simulink model "Powersystem_FMU"  (R2022a)
settings: Solver=ode23s  StartTime=0.0  StopTime=10  RelTol=1e-3
settings Model: Creator=au707539  LastModifiedBy=au528638
settings SolverCC: MaxZcPerStep=1

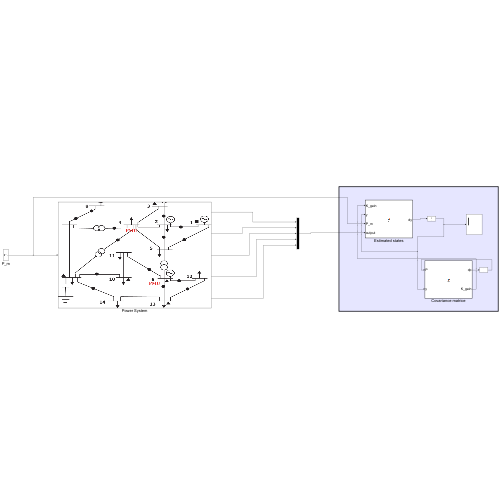
[thumbnail: Simulink's stored preview of the top-level diagram]
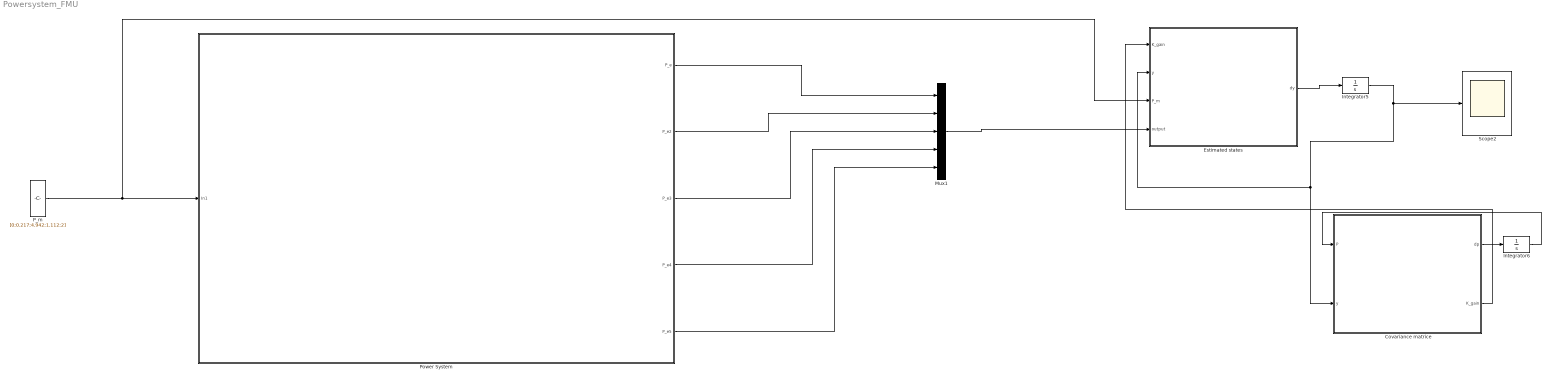
== system Powersystem_FMU ==
  Covariance matrice : MATLAB Function  TreatAsAtomicUnit=on
  Estimated states : MATLAB Function  TreatAsAtomicUnit=on
  Integrator5 : Integrator  InitialCondition=[1.07618884220704,1,0.179610235169918,1,-0.222670000000000,0.951,-0.152730000000000,0.91,-0.230910000000000,1]'
  Integrator6 : Integrator  InitialCondition=1*eye(10)
  Mux1 : Mux  Inputs=5
  P_m : Constant  Value=[0;0.217;4.942;1.112;2]
  Power System : Subsystem
      mask Display: image('IEEE.png'); % Use "Edit Image" on toolstrip to change.
  Scope2 : Scope
  wires:
  P_m/1 -> Estimated states/3(P_m), Power System/1(In1)
  Estimated states/1(dy) -> Integrator5/1
  Integrator5/1 -> Estimated states/2(y), Covariance matrice/2(y), Scope2/1
  Covariance matrice/1(dp) -> Integrator6/1
  Integrator6/1 -> Covariance matrice/1(P)
  Covariance matrice/2(K_gain) -> Estimated states/1(K_gain)
  Mux1/1 -> Estimated states/4(output)
  Power System/1(P_e) -> Mux1/1
  Power System/2(P_e2) -> Mux1/2
  Power System/3(P_e3) -> Mux1/3
  Power System/4(P_e4) -> Mux1/4
  Power System/5(P_e5) -> Mux1/5

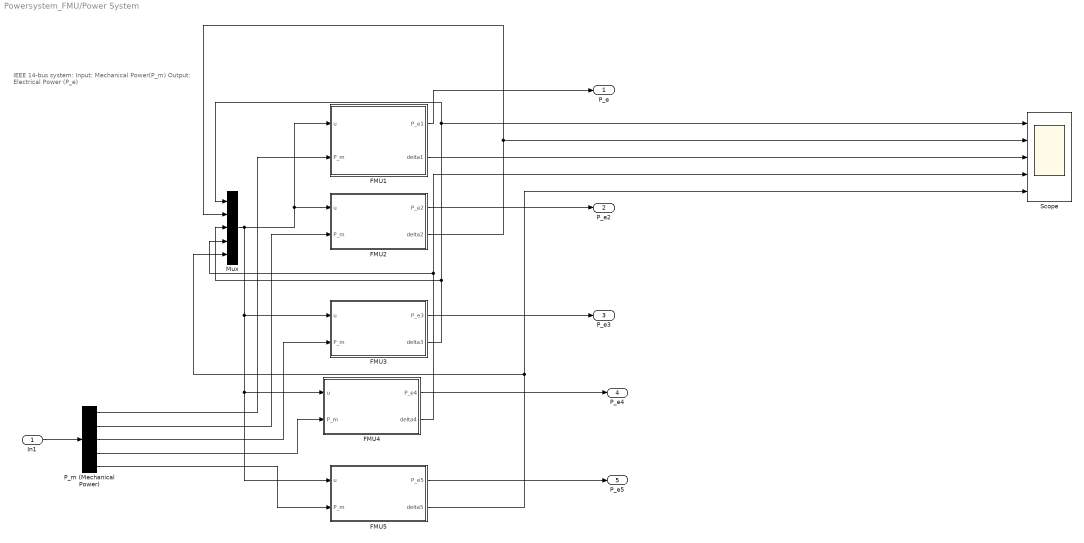
== system Powersystem_FMU/Power System ==
  note: IEEE 14-bus system:
      | Input: Mechanical Power(P_m)
      | Output: Electrical Power (P_e)
  In1 : Inport
  FMU1 : Subsystem
  FMU2 : Subsystem
  FMU3 : Subsystem
  FMU4 : Subsystem
  FMU5 : Subsystem
  Mux : Mux  Inputs=5
  P_m (Mechanical Power) : Demux  Outputs=5
  Scope : Scope  NumInputPorts=5
  P_e : Outport
  P_e2 : Outport  Port=2
  P_e3 : Outport  Port=3
  P_e4 : Outport  Port=4
  P_e5 : Outport  Port=5
  wires:
  FMU1/2(delta1) -> Scope/1, Mux/1
  FMU2/2(delta2) -> Scope/2, Mux/2
  In1/1 -> P_m (Mechanical Power)/1
  P_m (Mechanical Power)/1 -> FMU1/2(P_m)
  FMU1/1(P_e1) -> P_e/1
  P_m (Mechanical Power)/2 -> FMU2/2(P_m)
  FMU2/1(P_e2) -> P_e2/1
  P_m (Mechanical Power)/3 -> FMU3/2(P_m)
  FMU3/2(delta3) -> Scope/3, Mux/3
  FMU3/1(P_e3) -> P_e3/1
  P_m (Mechanical Power)/4 -> FMU4/2(P_m)
  FMU4/2(delta4) -> Scope/4, Mux/4
  FMU4/1(P_e4) -> P_e4/1
  P_m (Mechanical Power)/5 -> FMU5/2(P_m)
  FMU5/1(P_e5) -> P_e5/1
  FMU5/2(delta5) -> Mux/5, Scope/5
  Mux/1 -> FMU5/1(u), FMU4/1(u), FMU3/1(u), FMU2/1(u), FMU1/1(u)

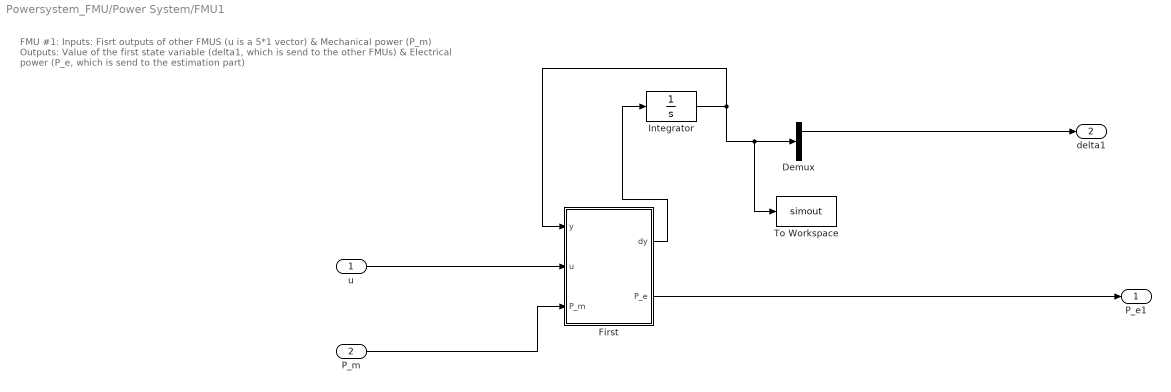
== system Powersystem_FMU/Power System/FMU1 ==
  note: FMU #1:
      | Inputs: Fisrt outputs of other FMUS (u is a 5*1 vector) & Mechanical power (P_m)
      | Outputs: Value of the first state variable (delta1, which is send to the other FMUs) & Electrical power (P_e, which is send to the estimation part)
  u : Inport
  P_m : Inport  Port=2
  Demux : Demux  Outputs=2
  First : MATLAB Function  TreatAsAtomicUnit=on
  Integrator : Integrator  InitialCondition=[1.0762;1]
  To Workspace : ToWorkspace  VariableName=simout  SaveFormat=Timeseries  SampleTime=-1
  P_e1 : Outport
  delta1 : Outport  Port=2
  wires:
  u/1 -> First/2(u)
  Integrator/1 -> First/1(y), To Workspace/1, Demux/1
  First/1(dy) -> Integrator/1
  P_m/1 -> First/3(P_m)
  First/2(P_e) -> P_e1/1
  Demux/1 -> delta1/1

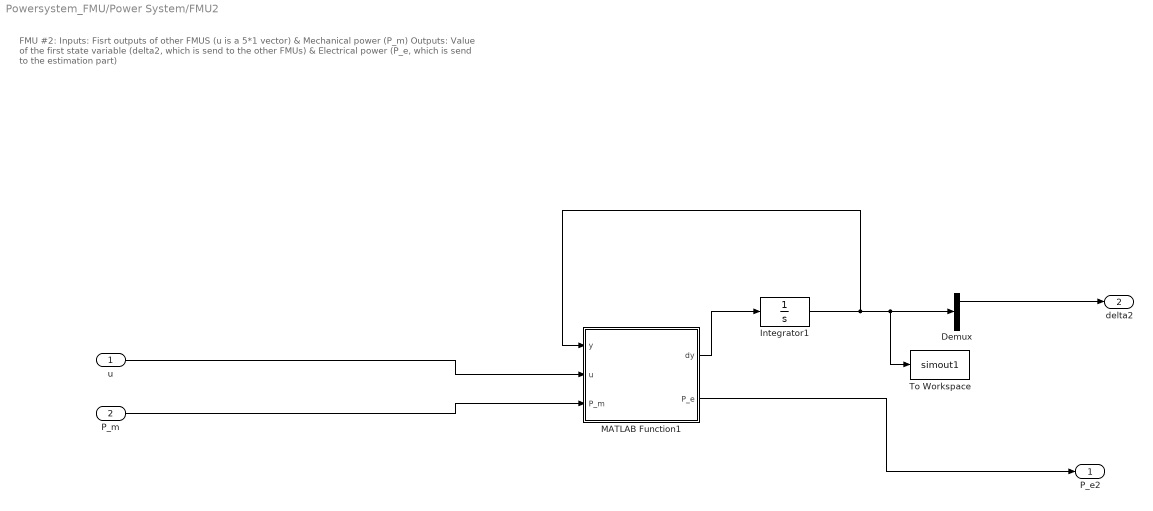
== system Powersystem_FMU/Power System/FMU2 ==
  note: FMU #2:
      | Inputs: Fisrt outputs of other FMUS (u is a 5*1 vector) & Mechanical power (P_m)
      | Outputs: Value of the first state variable (delta2, which is send to the other FMUs) & Electrical power (P_e, which is send to the estimation part)
  u : Inport
  P_m : Inport  Port=2
  Demux : Demux  Outputs=2
  Integrator1 : Integrator  InitialCondition=[0.1796;1]
  MATLAB Function1 : MATLAB Function  TreatAsAtomicUnit=on
  To Workspace : ToWorkspace  VariableName=simout1  SaveFormat=Timeseries  SampleTime=-1
  P_e2 : Outport
  delta2 : Outport  Port=2
  wires:
  P_m/1 -> MATLAB Function1/3(P_m)
  MATLAB Function1/1(dy) -> Integrator1/1
  u/1 -> MATLAB Function1/2(u)
  Integrator1/1 -> To Workspace/1, Demux/1, MATLAB Function1/1(y)
  Demux/1 -> delta2/1
  MATLAB Function1/2(P_e) -> P_e2/1

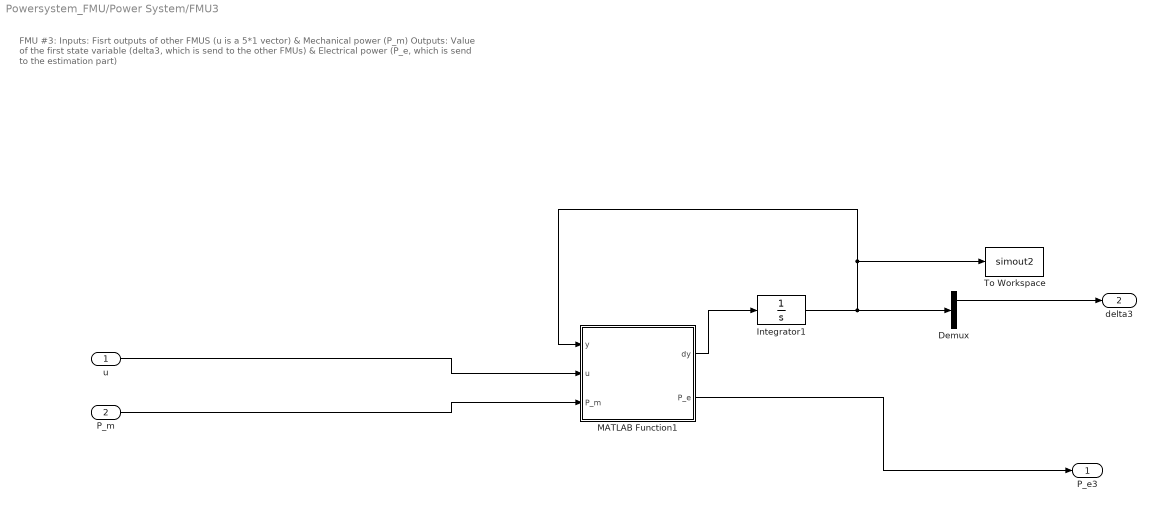
== system Powersystem_FMU/Power System/FMU3 ==
  note: FMU #3:
      | Inputs: Fisrt outputs of other FMUS (u is a 5*1 vector) & Mechanical power (P_m)
      | Outputs: Value of the first state variable (delta3, which is send to the other FMUs) & Electrical power (P_e, which is send to the estimation part)
  u : Inport
  P_m : Inport  Port=2
  Demux : Demux  Outputs=2
  Integrator1 : Integrator  InitialCondition=[0.1796;1]
  MATLAB Function1 : MATLAB Function  TreatAsAtomicUnit=on
  To Workspace : ToWorkspace  VariableName=simout2  SaveFormat=Timeseries  SampleTime=-1
  P_e3 : Outport
  delta3 : Outport  Port=2
  wires:
  P_m/1 -> MATLAB Function1/3(P_m)
  MATLAB Function1/1(dy) -> Integrator1/1
  u/1 -> MATLAB Function1/2(u)
  Integrator1/1 -> Demux/1, To Workspace/1, MATLAB Function1/1(y)
  Demux/1 -> delta3/1
  MATLAB Function1/2(P_e) -> P_e3/1

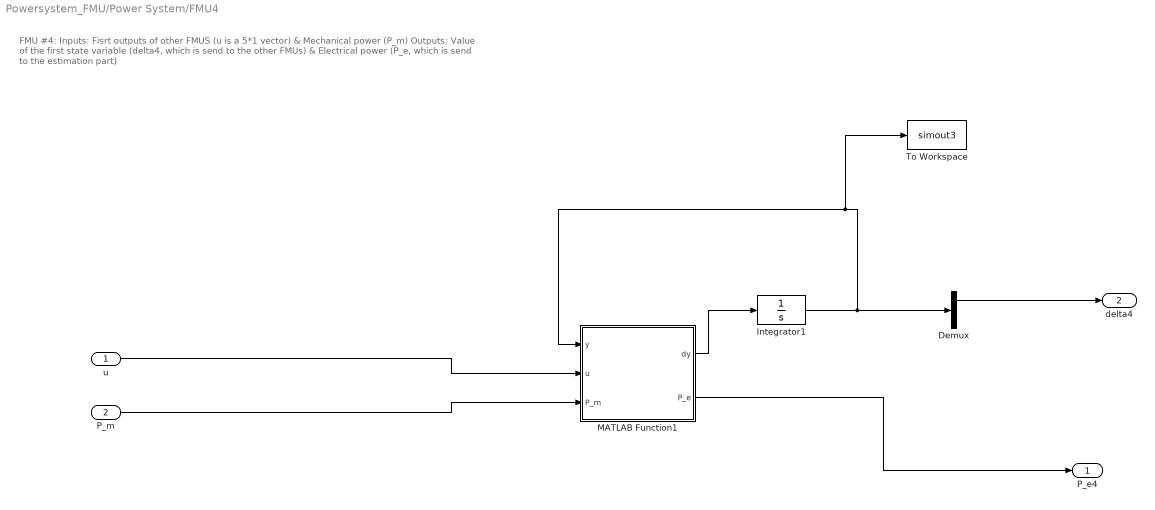
== system Powersystem_FMU/Power System/FMU4 ==
  note: FMU #4:
      | Inputs: Fisrt outputs of other FMUS (u is a 5*1 vector) & Mechanical power (P_m)
      | Outputs: Value of the first state variable (delta4, which is send to the other FMUs) & Electrical power (P_e, which is send to the estimation part)
  u : Inport
  P_m : Inport  Port=2
  Demux : Demux  Outputs=2
  Integrator1 : Integrator  InitialCondition=[0.1796;1]
  MATLAB Function1 : MATLAB Function  TreatAsAtomicUnit=on
  To Workspace : ToWorkspace  VariableName=simout3  SaveFormat=Timeseries  SampleTime=-1
  P_e4 : Outport
  delta4 : Outport  Port=2
  wires:
  P_m/1 -> MATLAB Function1/3(P_m)
  MATLAB Function1/1(dy) -> Integrator1/1
  u/1 -> MATLAB Function1/2(u)
  Demux/1 -> delta4/1
  MATLAB Function1/2(P_e) -> P_e4/1
  Integrator1/1 -> Demux/1, To Workspace/1, MATLAB Function1/1(y)

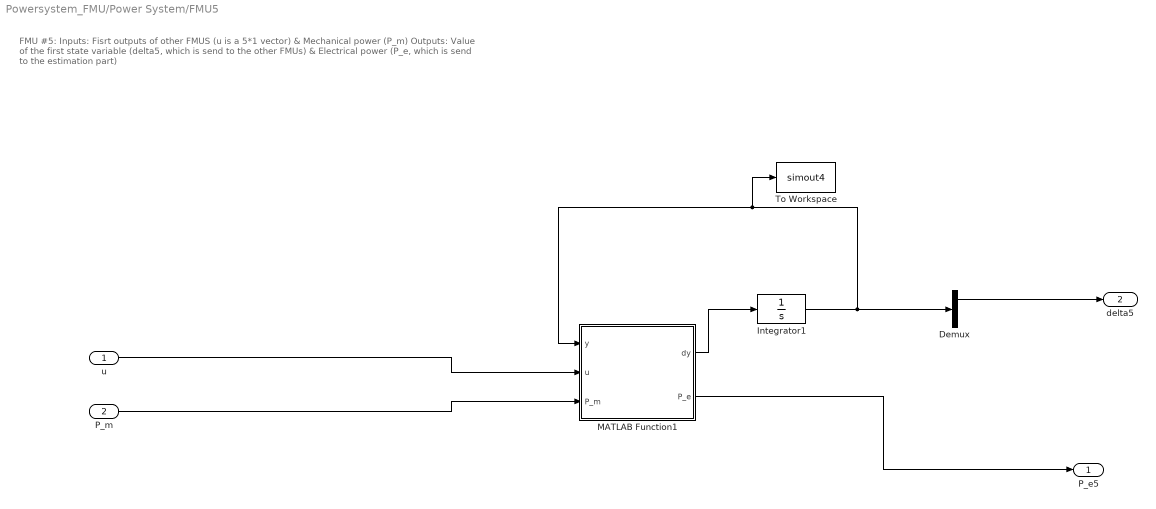
== system Powersystem_FMU/Power System/FMU5 ==
  note: FMU #5:
      | Inputs: Fisrt outputs of other FMUS (u is a 5*1 vector) & Mechanical power (P_m)
      | Outputs: Value of the first state variable (delta5, which is send to the other FMUs) & Electrical power (P_e, which is send to the estimation part)
  u : Inport
  P_m : Inport  Port=2
  Demux : Demux  Outputs=2
  Integrator1 : Integrator  InitialCondition=[0.1796;1]
  MATLAB Function1 : MATLAB Function  TreatAsAtomicUnit=on
  To Workspace : ToWorkspace  VariableName=simout4  SaveFormat=Timeseries  SampleTime=-1
  P_e5 : Outport
  delta5 : Outport  Port=2
  wires:
  P_m/1 -> MATLAB Function1/3(P_m)
  MATLAB Function1/1(dy) -> Integrator1/1
  u/1 -> MATLAB Function1/2(u)
  Integrator1/1 -> Demux/1, To Workspace/1, MATLAB Function1/1(y)
  Demux/1 -> delta5/1
  MATLAB Function1/2(P_e) -> P_e5/1

== matlab function Powersystem_FMU/Power System/FMU2/MATLAB Function1 ==
  data: y input; u input; dy output; P_m input; P_e output
%% This function formulates the dynamic model of the second synchronous machine in IEEE-14 bus test system
%% y is the state vector related to this Genrator, u is vector of all generators angles (delta), and P-m is Mechanical power injected to this machine
%% dy is the derivative of y which is calculated in this function and P-e is the electrical power which is calculated in this function
function [dy,P_e] = fcn(y,u,P_m)
dy=zeros(2,1);
P_e=0;
%%%%%%%Generators and network parameters (they can be defined as global
%%%%%%%parameters because they are fixed for all generators)%%%%%%%%%%%
N_SG=5;
X_d=[0.898 1.05 1.05 1.25 1.25];
Vol_mag=[1.06 1.045 1.01 1.011981 1.049336 1.016012 1.07 1.09 1.032756 1.03177 1.04708 1.053428 1.046967 1.020701];
P_Gen=[2.32 0.4 0 0 0];
Q_Gen=[0 0.424 0 0 0];
VOl_mag_Gen=[Vol_mag(1) Vol_mag(2) Vol_mag(3) Vol_mag(6) Vol_mag(8)];
M=[3.52e-3 0.436e-3 0.436e-3 1.406e-4 1.406e-4];
D=[2 2 2 2 2];
Y=[0.1017-2.4199i, 0.0096+0.9097i, -0.0567+0.5006i, -0.0322+0.4973i, -0.0186+0.5531i; 0.0096+0.9097i, 0.1375-3.5521i, -0.0574+0.9568i, -0.0437+0.8608i, ...
    -0.0395+0.8903i; -0.0567+0.5006i, -0.0574+0.9568i, 0.2630-2.9134i, -0.0640+0.8148i, -0.0791+0.6968i; -0.0322+0.4973i, -0.0437+0.8608i, -0.0640+0.8148i,...
    0.1156-3.0762i, 0.0303+0.9547i; -0.0186+0.5531i, -0.0395+0.8903i, -0.0791+0.6968i, 0.0303+0.9547i, 0.1117-3.0513i];
% [v_r, v_i]=pol2cart(Degrre_Gen,Vol_mag_Gen);

E_abs=zeros(5,1);
for i=1:5
    %     delta0(i)=angle(VOl_mag_Gen(i)+Q_Gen(i).*X_d(i)./VOl_mag_Gen(i) + 1i*P_Gen(i).*X_d(i)./VOl_mag_Gen(i))+Degrre_Gen(i);
    E_abs(i)=abs(VOl_mag_Gen(i)+Q_Gen(i).*X_d(i)./VOl_mag_Gen(i) + 1i*P_Gen(i).*X_d(i)./VOl_mag_Gen(i));
end
%%%%%%%%%%%%%%%%%%%%%%%%%%
delta=u(1:5);
sum1=0; %% local parameter
for j=1:N_SG

    sum1=sum1+E_abs(2)*E_abs(j)*abs(Y(2,j))*cos(delta(2)-delta(j)-angle(Y(2,j))); % All angles in Radian
end
P_e=sum1;

P_e=sum1;  % Second output (which is send to the estimation part)

dy(1)=y(2); %first entry of the function output

dy(2) =(1/M(2))*(P_m-P_e-D(2)*y(2));  %Second entry of the function output

== matlab function Powersystem_FMU/Power System/FMU1/First ==
  data: y input; u input; dy output; P_m input; P_e output
%% This function formulates the dynamic model of the first synchronous machine in IEEE-14 bus test system
%% y is the state vector related to this Genrator, u is vector of all generators angles (delta), and P-m is Mechanical power injected to this machine
%% dy is the derivative of y which is calculated in this function and P-e is the electrical power which is calculated in this function
function [dy,P_e] = fcn(y,u,P_m) 
dy=zeros(2,1);

%%%%%%%Generators and network parameters (they can be defined as global
%%%%%%%parameters because they are fixed for all generators)%%%%%%%%%%%%%
N_SG=5;
X_d=[0.898 1.05 1.05 1.25 1.25];
Vol_mag=[1.06 1.045 1.01 1.011981 1.049336 1.016012 1.07 1.09 1.032756 1.03177 1.04708 1.053428 1.046967 1.020701];
P_Gen=[2.32 0.4 0 0 0];
Q_Gen=[0 0.424 0 0 0];
VOl_mag_Gen=[Vol_mag(1) Vol_mag(2) Vol_mag(3) Vol_mag(6) Vol_mag(8)];
M=[3.52e-3 0.436e-3 0.436e-3 1.406e-4 1.406e-4];
D=[2 2 2 2 2];
Y=[0.1017-2.4199i, 0.0096+0.9097i, -0.0567+0.5006i, -0.0322+0.4973i, -0.0186+0.5531i; 0.0096+0.9097i, 0.1375-3.5521i, -0.0574+0.9568i, -0.0437+0.8608i, ...
    -0.0395+0.8903i; -0.0567+0.5006i, -0.0574+0.9568i, 0.2630-2.9134i, -0.0640+0.8148i, -0.0791+0.6968i; -0.0322+0.4973i, -0.0437+0.8608i, -0.0640+0.8148i,...
    0.1156-3.0762i, 0.0303+0.9547i; -0.0186+0.5531i, -0.0395+0.8903i, -0.0791+0.6968i, 0.0303+0.9547i, 0.1117-3.0513i];
% [v_r, v_i]=pol2cart(Degrre_Gen,Vol_mag_Gen);

E_abs=zeros(5,1); %local parameter
for i=1:5
    %     delta0(i)=angle(VOl_mag_Gen(i)+Q_Gen(i).*X_d(i)./VOl_mag_Gen(i) + 1i*P_Gen(i).*X_d(i)./VOl_mag_Gen(i))+Degrre_Gen(i);
    E_abs(i)=abs(VOl_mag_Gen(i)+Q_Gen(i).*X_d(i)./VOl_mag_Gen(i) + 1i*P_Gen(i).*X_d(i)./VOl_mag_Gen(i));
end
%%%%%%%%%%%%%%%%%%%%%%%%%%
delta=u(1:5);
sum1=0; %% local parameter
for j=1:N_SG

    sum1=sum1+E_abs(1)*E_abs(j)*abs(Y(1,j))*cos(delta(1)-delta(j)-angle(Y(1,j))); % All angles in Radian
end

P_e=sum1;  % Second output (which is send to the estimation part)

dy(1)=y(2); %first entry of the function output

dy(2) =(1/M(1))*(P_m-P_e-D(1)*y(2)); %Second entry of the function output

== matlab function Powersystem_FMU/Power System/FMU4/MATLAB Function1 ==
  data: y input; u input; dy output; P_m input; P_e output
%% This function formulates the dynamic model of the fourth synchronous machine in IEEE-14 bus test system
%% y is the state vector related to this Genrator, u is vector of all generators angles (delta), and P-m is Mechanical power injected to this machine
%% dy is the derivative of y which is calculated in this function and P-e is the electrical power which is calculated in this function
function [dy,P_e] = fcn(y,u,P_m)
dy=zeros(2,1);
P_e=0;
%%%%%%%Generators and network parameters (they can be defined as global
%%%%%%%parameters because they are fixed for all generators)%%%%%%%%%%%
N_SG=5;
X_d=[0.898 1.05 1.05 1.25 1.25];
Vol_mag=[1.06 1.045 1.01 1.011981 1.049336 1.016012 1.07 1.09 1.032756 1.03177 1.04708 1.053428 1.046967 1.020701];
P_Gen=[2.32 0.4 0 0 0];
Q_Gen=[0 0.424 0 0 0];
VOl_mag_Gen=[Vol_mag(1) Vol_mag(2) Vol_mag(3) Vol_mag(6) Vol_mag(8)];
M=[3.52e-3 0.436e-3 0.436e-3 1.406e-4 1.406e-4];
D=[2 2 2 2 2];
Y=[0.1017-2.4199i, 0.0096+0.9097i, -0.0567+0.5006i, -0.0322+0.4973i, -0.0186+0.5531i; 0.0096+0.9097i, 0.1375-3.5521i, -0.0574+0.9568i, -0.0437+0.8608i, ...
    -0.0395+0.8903i; -0.0567+0.5006i, -0.0574+0.9568i, 0.2630-2.9134i, -0.0640+0.8148i, -0.0791+0.6968i; -0.0322+0.4973i, -0.0437+0.8608i, -0.0640+0.8148i,...
    0.1156-3.0762i, 0.0303+0.9547i; -0.0186+0.5531i, -0.0395+0.8903i, -0.0791+0.6968i, 0.0303+0.9547i, 0.1117-3.0513i];
% [v_r, v_i]=pol2cart(Degrre_Gen,Vol_mag_Gen);

E_abs=zeros(5,1);
for i=1:5
    %     delta0(i)=angle(VOl_mag_Gen(i)+Q_Gen(i).*X_d(i)./VOl_mag_Gen(i) + 1i*P_Gen(i).*X_d(i)./VOl_mag_Gen(i))+Degrre_Gen(i);
    E_abs(i)=abs(VOl_mag_Gen(i)+Q_Gen(i).*X_d(i)./VOl_mag_Gen(i) + 1i*P_Gen(i).*X_d(i)./VOl_mag_Gen(i));
end
%%%%%%%%%%%%%%%%%%%%%%%%%%
delta=u(1:5);
sum1=0; %% local parameter
for j=1:N_SG

    sum1=sum1+E_abs(4)*E_abs(j)*abs(Y(4,j))*cos(delta(4)-delta(j)-angle(Y(4,j))); % All angles in Radian
end

P_e=sum1;

P_e=sum1;  % Second output (which is send to the estimation part)

dy(1)=y(2); %first entry of the function output

dy(2) =(1/M(4))*(P_m-P_e-D(4)*y(2));  %Second entry of the function output

== matlab function Powersystem_FMU/Power System/FMU5/MATLAB Function1 ==
  data: y input; u input; dy output; P_m input; P_e output
%% This function formulates the dynamic model of the fifth synchronous machine in IEEE-14 bus test system
%% y is the state vector related to this Genrator, u is vector of all generators angles (delta), and P-m is Mechanical power injected to this machine
%% dy is the derivative of y which is calculated in this function and P-e is the electrical power which is calculated in this function
function [dy,P_e] = fcn(y,u,P_m)
dy=zeros(2,1);
P_e=0;
%%%%%%%Generators and network parameters (they can be defined as global
%%%%%%%parameters because they are fixed for all generators)%%%%%%%%%%%
N_SG=5;
X_d=[0.898 1.05 1.05 1.25 1.25];
Vol_mag=[1.06 1.045 1.01 1.011981 1.049336 1.016012 1.07 1.09 1.032756 1.03177 1.04708 1.053428 1.046967 1.020701];
P_Gen=[2.32 0.4 0 0 0];
Q_Gen=[0 0.424 0 0 0];
VOl_mag_Gen=[Vol_mag(1) Vol_mag(2) Vol_mag(3) Vol_mag(6) Vol_mag(8)];
M=[3.52e-3 0.436e-3 0.436e-3 1.406e-4 1.406e-4];
D=[2 2 2 2 2];
Y=[0.1017-2.4199i, 0.0096+0.9097i, -0.0567+0.5006i, -0.0322+0.4973i, -0.0186+0.5531i; 0.0096+0.9097i, 0.1375-3.5521i, -0.0574+0.9568i, -0.0437+0.8608i, ...
    -0.0395+0.8903i; -0.0567+0.5006i, -0.0574+0.9568i, 0.2630-2.9134i, -0.0640+0.8148i, -0.0791+0.6968i; -0.0322+0.4973i, -0.0437+0.8608i, -0.0640+0.8148i,...
    0.1156-3.0762i, 0.0303+0.9547i; -0.0186+0.5531i, -0.0395+0.8903i, -0.0791+0.6968i, 0.0303+0.9547i, 0.1117-3.0513i];
% [v_r, v_i]=pol2cart(Degrre_Gen,Vol_mag_Gen);

E_abs=zeros(5,1);
for i=1:5
    %     delta0(i)=angle(VOl_mag_Gen(i)+Q_Gen(i).*X_d(i)./VOl_mag_Gen(i) + 1i*P_Gen(i).*X_d(i)./VOl_mag_Gen(i))+Degrre_Gen(i);
    E_abs(i)=abs(VOl_mag_Gen(i)+Q_Gen(i).*X_d(i)./VOl_mag_Gen(i) + 1i*P_Gen(i).*X_d(i)./VOl_mag_Gen(i));
end
%%%%%%%%%%%%%%%%%%%%%%%%%%
delta=u(1:5);
sum1=0; %% local parameter
for j=1:N_SG

    sum1=sum1+E_abs(5)*E_abs(j)*abs(Y(5,j))*cos(delta(5)-delta(j)-angle(Y(5,j))); % All angles in Radian
end

P_e=sum1;

P_e=sum1;  % Second output (which is send to the estimation part)

dy(1)=y(2); %first entry of the function output

dy(2) =(1/M(5))*(P_m-P_e-D(5)*y(2));  %Second entry of the function output

== matlab function Powersystem_FMU/Estimated states ==
  data: K_gain input; dy output; y input; P_m input; output input
function dy = fcn(K_gain,y,P_m,output)
dy=zeros(10,1); %Number of states=number of generators*Order of model+ number of elements of matrix P (10*10)

N_SG=5; % Number of generators in the grid
estimatedOutput=zeros(5,1);
%Load flow results for IEEE 14 bus system

X_d=[0.898 1.05 1.05 1.25 1.25];
Angle_rad=[0 -0.0871 -0.22267 -0.1785 -0.23091 -0.15273 -0.25161 -0.23091 -0.25853 -0.26223 -0.25897 -0.26645 -0.2671 -0.28018];%% Bus voltage phases (all are in rad)
Vol_mag=[1.06 1.045 1.01 1.011981 1.049336 1.016012 1.07 1.09 1.032756 1.03177 1.04708 1.053428 1.046967 1.020701];%% Bus voltage magnitudes
P_Gen=[2.32 0.4 0 0 0]; % Active power
Q_Gen=[0 0.424 0 0 0]; % Reactive Power
VOl_mag_Gen=[Vol_mag(1) Vol_mag(2) Vol_mag(3) Vol_mag(6) Vol_mag(8)];
Phase_Gen=[Angle_rad(1) Angle_rad(2) Angle_rad(3) Angle_rad(6) Angle_rad(8)];
% [v_r, v_i]=pol2cart(Degrre_Gen,Vol_mag_Gen);

%%Calculating the phases and magnitudes of the generator voltages
delta0=zeros(5,1);
E_abs=zeros(5,1);
for i=1:5
    delta0(i)=angle(VOl_mag_Gen(i)+Q_Gen(i).*X_d(i)./VOl_mag_Gen(i) + 1i*P_Gen(i).*X_d(i)./VOl_mag_Gen(i))+Phase_Gen(i);
    E_abs(i)=abs(VOl_mag_Gen(i)+Q_Gen(i).*X_d(i)./VOl_mag_Gen(i) + 1i*P_Gen(i).*X_d(i)./VOl_mag_Gen(i));
end

% Reduced admittance matrix (all in p.u.)
Y_red=[0.1017-2.4199i, 0.0096+0.9097i, -0.0567+0.5006i, -0.0322+0.4973i, -0.0186+0.5531i; 0.0096+0.9097i, 0.1375-3.5521i, -0.0574+0.9568i, -0.0437+0.8608i, ...
    -0.0395+0.8903i; -0.0567+0.5006i, -0.0574+0.9568i, 0.2630-2.9134i, -0.0640+0.8148i, -0.0791+0.6968i; -0.0322+0.4973i, -0.0437+0.8608i, -0.0640+0.8148i,...
    0.1156-3.0762i, 0.0303+0.9547i; -0.0186+0.5531i, -0.0395+0.8903i, -0.0791+0.6968i, 0.0303+0.9547i, 0.1117-3.0513i];

%---------------------------------------------------------------------------------------------------------------------------------------

% Define simulation parameters
% Omega_s=2*pi*50;
% Define M as rotor inertia constant (should be a vector of size N_SG)
H=[5.184 6.54 6.54 5.06 5.06];
S_bas=100;
f_s=50;
M=[3.52e-3 0.436e-3 0.436e-3 1.406e-4 1.406e-4];
% Define K_D as damping factor (should be a vector of size N_SG)
D=[2 2 2 2 2];
% K_D=D/Omega_s;
% T_d0prime as open-circuit time constant for d-axis of SG (size N_SG)
% T_d0prime=8;
% 
% % Define Machine Parameters
% X_d=0.2;
% Xprime_d=0.033;


% Initialization 
P_e=zeros(5,1);  % Electrical Power



%%% calculating the estimated output
for i=1:5
     sum1=0;
    for j=1:5
       
        sum1=sum1+E_abs(i)*E_abs(j)*abs(Y_red(i,j))*cos(y(2*i-1)-y(2*j-1)-angle(Y_red(i,j))); % All angles in Radian
    end
    estimatedOutput(i)=sum1;
end


for i=1:N_SG
    %%Dynamic equation of voltage angles of generators
    %delta_dot(i)=Omega_s*(Omega(i)-1);
    dy(2*i-1)=y(2*i)+K_gain(2*i-1,:)*(output-estimatedOutput);

    sum1=0;
    for j=1:N_SG
       
        sum1=sum1+E_abs(i)*E_abs(j)*abs(Y_red(i,j))*cos(y(2*i-1)-y(2*j-1)-angle(Y_red(i,j))); % All angles in Radian
    end
    P_e(i)=sum1;
    
    %Omega_dot(i)=(Omega_s/M(i))*(P_m(i)-P_e(i)-K_D(i)*(Omega(i)-1)); % P_m is the mechanical input
    dy(2*i)=(1/M(i))*(P_m(i)-P_e(i)-D(i)*y(2*i))+K_gain(2*i,:)*(output-estimatedOutput);
end

== matlab function Powersystem_FMU/Covariance matrice ==
  data: dp output; P input; K_gain output; y input
function [dp,K_gain] = fcn(P,y)
dp=zeros(10,10); %Number of states=number of generators*Order of model+ number of elements of matrix P (10*10)

N_SG=5; % Number of generators in the grid
estimatedOutput=zeros(5,1);
%Load flow results for IEEE 14 bus system

X_d=[0.898 1.05 1.05 1.25 1.25];
Angle_rad=[0 -0.0871 -0.22267 -0.1785 -0.23091 -0.15273 -0.25161 -0.23091 -0.25853 -0.26223 -0.25897 -0.26645 -0.2671 -0.28018];%% Bus voltage phases (all are in rad)
Vol_mag=[1.06 1.045 1.01 1.011981 1.049336 1.016012 1.07 1.09 1.032756 1.03177 1.04708 1.053428 1.046967 1.020701];%% Bus voltage magnitudes
P_Gen=[2.32 0.4 0 0 0]; % Active power
Q_Gen=[0 0.424 0 0 0]; % Reactive Power
VOl_mag_Gen=[Vol_mag(1) Vol_mag(2) Vol_mag(3) Vol_mag(6) Vol_mag(8)];
Phase_Gen=[Angle_rad(1) Angle_rad(2) Angle_rad(3) Angle_rad(6) Angle_rad(8)];
% [v_r, v_i]=pol2cart(Degrre_Gen,Vol_mag_Gen);

%%Calculating the phases and magnitudes of the generator voltages
delta0=zeros(5,1);
E_abs=zeros(5,1);
for i=1:5
    delta0(i)=angle(VOl_mag_Gen(i)+Q_Gen(i).*X_d(i)./VOl_mag_Gen(i) + 1i*P_Gen(i).*X_d(i)./VOl_mag_Gen(i))+Phase_Gen(i);
    E_abs(i)=abs(VOl_mag_Gen(i)+Q_Gen(i).*X_d(i)./VOl_mag_Gen(i) + 1i*P_Gen(i).*X_d(i)./VOl_mag_Gen(i));
end

% Reduced admittance matrix (all in p.u.)
Y_red=[0.1017-2.4199i, 0.0096+0.9097i, -0.0567+0.5006i, -0.0322+0.4973i, -0.0186+0.5531i; 0.0096+0.9097i, 0.1375-3.5521i, -0.0574+0.9568i, -0.0437+0.8608i, ...
    -0.0395+0.8903i; -0.0567+0.5006i, -0.0574+0.9568i, 0.2630-2.9134i, -0.0640+0.8148i, -0.0791+0.6968i; -0.0322+0.4973i, -0.0437+0.8608i, -0.0640+0.8148i,...
    0.1156-3.0762i, 0.0303+0.9547i; -0.0186+0.5531i, -0.0395+0.8903i, -0.0791+0.6968i, 0.0303+0.9547i, 0.1117-3.0513i];

%---------------------------------------------------------------------------------------------------------------------------------------

% Define simulation parameters
% Omega_s=2*pi*50;
% Define M as rotor inertia constant (should be a vector of size N_SG)
H=[5.184 6.54 6.54 5.06 5.06];
S_bas=100;
f_s=50;
M=[3.52e-3 0.436e-3 0.436e-3 1.406e-4 1.406e-4];
% Define K_D as damping factor (should be a vector of size N_SG)
D=[2 2 2 2 2];
% K_D=D/Omega_s;
% T_d0prime as open-circuit time constant for d-axis of SG (size N_SG)
% T_d0prime=8;
% 
% % Define Machine Parameters
% X_d=0.2;
% Xprime_d=0.033;

% Define inputs of the system P_m(i) & E_f(i)

P_m=[0 0.217 0.942 0.112 0];

% Initialization 
P_e=zeros(5,1);  % Electrical Power

sigma=1e-2;  % variance
Q=sigma^2*eye(10); %Process noise covariance matrix
R=sigma^2*eye(5); %Measurement noise covariance matrix

% Computing partial derivetive matrices
L=eye(10);
M_p=eye(5);
C=zeros(5,10);
A=zeros(10,10);
% y=[1.07618884220704,1,0.179610235169918,1,-0.222670000000000,1,-0.152730000000000,1,-0.230910000000000,1]';

for j=1:5
    A(2*j-1,:)=0;
    A(2*j-1,2*j)=1;
    for i=1:10
        if i==2*j
            A(2*j,i)=-D(j)/M(j);
        elseif i==2*j-1
            sum=0;
            for k=1:5
                if k~=j
                    sum=sum+(1/M(j))*(E_abs(j)*E_abs(k)*abs(Y_red(j,k))*sin(y(2*j-1)-y(2*k-1)-angle(Y_red(j,k))));
                else
                    sum=sum;
                end          
            A(2*j,i)=sum;
            end
        elseif rem(i,2)==0
            A(2*j,i)=0;
        else
            A(2*j,i)=-(1/M(j))*E_abs(j)*E_abs((i+1)/2)*abs(Y_red(j,(i+1)/2))*sin(y(2*j-1)-y(2*((i+1)/2)-1)-angle(Y_red(j,(i+1)/2)));
        end
    end
end


for j=1:5
    for i=1:10
        if i==2*j-1
            sum=0;
            for k=1:5
                if k~=j
                    sum=sum-(1/M(j))*(E_abs(j)*E_abs(k)*abs(Y_red(j,k))*sin(y(2*j-1)-y(2*k-1)-angle(Y_red(j,k))));
                else
                    sum=sum;
                end          
            C(j,i)=sum;
            end
        elseif rem(i,2)==0
            C(j,i)=0;
        else
            C(j,i)=E_abs(j)*E_abs((i+1)/2)*abs(Y_red(j,(i+1)/2))*sin(y(2*j-1)-y(2*((i+1)/2)-1)-angle(Y_red(j,(i+1)/2)));
        end
    end
end

Q_tilda=L*Q*L';
R_tilda=M_p*R*M_p';


K_gain=P*C'*R_tilda^-1; % Kalman gain


  
 % dynamic equation of P
  dp=A*P+P*A'+Q_tilda-P*C'*(R_tilda^-1)*C*P;

== matlab function Powersystem_FMU/Power System/FMU3/MATLAB Function1 ==
  data: y input; u input; dy output; P_m input; P_e output
%% This function formulates the dynamic model of the third synchronous machine in IEEE-14 bus test system
%% y is the state vector related to this Genrator, u is vector of all generators angles (delta), and P-m is Mechanical power injected to this machine
%% dy is the derivative of y which is calculated in this function and P-e is the electrical power which is calculated in this function
function [dy,P_e] = fcn(y,u,P_m) 
dy=zeros(2,1);
P_e=0;
%%%%%%%Generators and network parameters (they can be defined as global
%%%%%%%parameters because they are fixed for all generators)%%%%%%%%%%%
N_SG=5;
X_d=[0.898 1.05 1.05 1.25 1.25];
Vol_mag=[1.06 1.045 1.01 1.011981 1.049336 1.016012 1.07 1.09 1.032756 1.03177 1.04708 1.053428 1.046967 1.020701];
P_Gen=[2.32 0.4 0 0 0];
Q_Gen=[0 0.424 0 0 0];
VOl_mag_Gen=[Vol_mag(1) Vol_mag(2) Vol_mag(3) Vol_mag(6) Vol_mag(8)];
M=[3.52e-3 0.436e-3 0.436e-3 1.406e-4 1.406e-4];
D=[2 2 2 2 2];
Y=[0.1017-2.4199i, 0.0096+0.9097i, -0.0567+0.5006i, -0.0322+0.4973i, -0.0186+0.5531i; 0.0096+0.9097i, 0.1375-3.5521i, -0.0574+0.9568i, -0.0437+0.8608i, ...
    -0.0395+0.8903i; -0.0567+0.5006i, -0.0574+0.9568i, 0.2630-2.9134i, -0.0640+0.8148i, -0.0791+0.6968i; -0.0322+0.4973i, -0.0437+0.8608i, -0.0640+0.8148i,...
    0.1156-3.0762i, 0.0303+0.9547i; -0.0186+0.5531i, -0.0395+0.8903i, -0.0791+0.6968i, 0.0303+0.9547i, 0.1117-3.0513i];
% [v_r, v_i]=pol2cart(Degrre_Gen,Vol_mag_Gen);

E_abs=zeros(5,1);
for i=1:5
    %     delta0(i)=angle(VOl_mag_Gen(i)+Q_Gen(i).*X_d(i)./VOl_mag_Gen(i) + 1i*P_Gen(i).*X_d(i)./VOl_mag_Gen(i))+Degrre_Gen(i);
    E_abs(i)=abs(VOl_mag_Gen(i)+Q_Gen(i).*X_d(i)./VOl_mag_Gen(i) + 1i*P_Gen(i).*X_d(i)./VOl_mag_Gen(i));
end
%%%%%%%%%%%%%%%%%%%%%%%%%%
delta=u(1:5);
sum1=0; %% local parameter
for j=1:N_SG

    sum1=sum1+E_abs(3)*E_abs(j)*abs(Y(3,j))*cos(delta(3)-delta(j)-angle(Y(3,j))); % All angles in Radian
end

P_e=sum1;

P_e=sum1;  % Second output (which is send to the estimation part)

dy(1)=y(2); %first entry of the function output

dy(2) =(1/M(3))*(P_m-P_e-D(3)*y(2));  %Second entry of the function output
